simulink model "week7_fuzzy"  (R2019a)
settings: Solver=VariableStepAuto  StartTime=0.0  StopTime=200  RelTol=1e-3
libraries: fuzblock x1
settings Model: Creator=ASUS  LastModifiedBy=ASUS
settings DataIOCC: ReturnWorkspaceOutputs=off

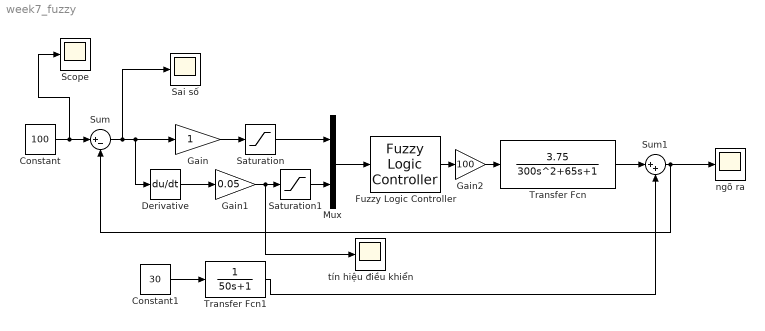
== system week7_fuzzy ==
  Constant : Constant  Value=100
  Constant1 : Constant  Value=30
  Derivative : Derivative
  Fuzzy Logic Controller : fuzblock/Fuzzy Logic  Controller  FIS='fuzzy_nhiet'  OutputSampleNumber=101  DataType=double  FuzzifiedInputs=off  RuleFiringStrengths=off  RuleOutputs=off  AggregatedOutputs=off  SimulateUsing=Interpreted execution  OutOfRangeInputValueMessage=warning  NoRuleFiredMessage=warning  EmptyOutputFuzzySetMessage=warning
  Gain : Gain
  Gain1 : Gain  Gain=0.05
  Gain2 : Gain  Gain=100
  Mux : Mux  Inputs=2
  "Sai số " : Scope
  Saturation : Saturate  UpperLimit=1  LowerLimit=-1
  Saturation1 : Saturate  UpperLimit=1  LowerLimit=-1
  Scope : Scope
  Sum : Sum  Inputs=|+-
  Sum1 : Sum  Inputs=|++
  Transfer Fcn : TransferFcn  Numerator=[3.75]  Denominator=[300 65 1]
  Transfer Fcn1 : TransferFcn  Denominator=[50 1]
  ngõ ra : Scope
  tín hiệu điều khiển : Scope
  wires:
  Gain2/1 -> Transfer Fcn/1
  Mux/1 -> Fuzzy Logic Controller/1
  Fuzzy Logic Controller/1 -> Gain2/1
  Derivative/1 -> Gain1/1
  Sum/1 -> "Sai số "/1, Derivative/1, Gain/1
  Constant/1 -> Scope/1, Sum/1
  Constant1/1 -> Transfer Fcn1/1
  Transfer Fcn/1 -> Sum1/1
  Sum1/1 -> ngõ ra/1, Sum/2
  Transfer Fcn1/1 -> Sum1/2
  Gain/1 -> Saturation/1
  Saturation/1 -> Mux/1
  Gain1/1 -> tín hiệu điều khiển/1, Saturation1/1
  Saturation1/1 -> Mux/2
